simulink model "QPSK_synch_baseband"  (R2024a)
settings: Solver=VariableStepDiscrete  StartTime=0.0  StopTime=500000/fs  RelTol=1e-3  EnableMultiTasking=on
values from neighbouring files (symbols this model uses):
  fs = 50e6    (= 50000000)    [test.m]    (also in workspaceLoader.m = 75000000)
  K1 = (4*d*Bn*ts)/(Ko*Kp*(d+1/(4*d)))    (= 0.0399959725225)    [test.m]
  K2 = (4*(Bn*ts)^2)/(Ko*Kp*(d+1/4*d)^2)    (= 0.0011523480091)    [test.m]
  Ko = 1    [test.m]
undefined symbols (not defined in the file or in its folder): startfcn_constellation
libraries: dspfdesign x2, commfilt2 x2, dspsigops x2
CloseFcn:
  | closefcn_model;
Description:
  | Software, Simulation Examples and Design Exercises Licence Agreement
  | 
  | This license agreement refers to the simulation examples, design exercises and files,
  | and associated software MATLAB and Simulink resources that accompany the book:
  | 
  |      Title: Software Defined Radio using MATLAB & Simulink and the RTL-SDR
  |      Published by Strathclyde Academic Media, 2015
  |      Authored by Robert W. Stewart, Kenneth W. Barlee, Dale S.W. Atkinson,
  |      and Louise H. Crockett
  | 
  | and made available as a download from, www.desktopSDR.com or variously acquired
  | by other means such as via USB storage, cloud storage, disk or any other electronic
  | or optical or magnetic storage mechanism. These files and associated software may
  | be used subject to the terms of agreement of the conditions below:
  | 
  |     Copyright © 2015 Robert W. Stewart, Kenneth W. Barlee, Dale S.W. Atkinson,
  |     and Louise H. Crockett
  |     All rights reserved.
  | 
  | Redistribution and use in source and binary forms, with or without modification, are
  | permitted provided that the following conditions are met:
  | 
  |    1.  Redistributions of source code must retain the above copyright notice, this list of
  |         conditions and the following disclaimer.
  | 
  |    2.  Redistributions in binary form must reproduce the above copyright notice, this
  |         list of conditions and the following disclaimer in the documentation and/or other
  |         materials provided with the distribution.
  | 
  |    3.  Neither the name of the copyright holder nor the names of its contributors may
  |         be used to endorse or promote products derived from this software without
  |         specific prior written permission.
  | 
  |    4.  In all cases, the software is, and all modifications and derivatives of the
  |         software shall be, licensed to you solely for use in conjunction with The
  |         MathWorks, Inc. products and service offerings.
  | 
  | THIS SOFTWARE IS PROVIDED BY THE COPYRIGHT HOLDERS AND CONTRIBUTORS
  | "AS IS" AND ANY EXPRESS OR IMPLIED WARRANTIES, INCLUDING, BUT NOT LIMITED
  | TO, THE IMPLIED WARRANTIES OF MERCHANTABILITY AND FITNESS FOR A
  | PARTICULAR PURPOSE ARE DISCLAIMED. IN NO EVENT SHALL THE COPYRIGHT
  | HOLDER OR CONTRIBUTORS BE LIABLE FOR ANY DIRECT, INDIRECT, INCIDENTAL,
  | SPECIAL, EXEMPLARY, OR CONSEQUENTIAL DAMAGES (INCLUDING, BUT NOT
  | LIMITED TO, PROCUREMENT OF SUBSTITUTE GOODS OR SERVICES; LOSS OF USE,
  | DATA, OR PROFITS; OR BUSINESS INTERRUPTION) HOWEVER CAUSED AND ON ANY
  | THEORY OF LIABILITY, WHETHER IN CONTRACT, STRICT LIABILITY, OR TORT
  | (INCLUDING NEGLIGENCE OR OTHERWISE) ARISING IN ANY WAY OUT OF THE USE
  | OF THIS SOFTWARE, EVEN IF ADVISED OF THE POSSIBILITY OF SUCH DAMAGE.
  | 
  | 
  | Audio Tracks used in Simulations Examples and Design Exercises
  | 
  | The music and vocal files used within the Examples files and software within the book
  | were variously written, arranged, performed, recorded and produced by Garrey Rice,
  | Adam Struth, Jamie Struth, Iain Thistlethwaite and also Marshall Craigmyle who
  | collectively, and individually where appropriate, assert and retain all of their copyright,
  | performance and artistic rights. Permission to use and reproduce this music is
  | granted for all purposes associated with MATLAB and Simulink software and the
  | simulation examples and design exercises files that accompany this book. Requests to
  | use the music for any other purpose should be directed to: info@desktopSDR.com.
  | For information on music track names, full credits, and links to the musicians please
  | refer to www.desktopSDR.com/more/audio.
settings Model: Creator=desktopSDR Team  LastModifiedBy=admin
settings SolverCC: AlgebraicLoopSolver=TrustRegion
settings DataIOCC: SaveFormat=Array  SaveOutput=off  SignalLogging=off  SaveTime=off  ReturnWorkspaceOutputs=off
settings OptimizationCC: LifeSpan=inf
settings DebuggingCC: UnderspecifiedInitializationDetection=Classic  MergeDetectMultiDrivingBlocksExec=none  SolverPrmCheckMsg=warning  UnconnectedInputMsg=warning  UnconnectedOutputMsg=warning  UnconnectedLineMsg=warning  SFUnexpectedBacktrackingDiag=warning  SFNoUnconditionalDefaultTransitionDiag=warning  SFExecutionAtInitializationDiag=none  ArithmeticOperatorsInVariantConditions=warning
settings HardwareCC: ProdBitPerPointer=32  ProdBitPerSizeT=32  ProdBitPerPtrDiffT=32  ProdLargestAtomicFloat=None  ProdIntDivRoundTo=Undefined  ProdEndianess=Unspecified  ProdWordSize=32  ProdHWDeviceType=32-bit Generic
settings ModelReferenceCC: PropagateSignalLabelsOutOfModel=off
settings SFSimCC: SimUseLocalCustomCode=off  CustomCodeUndefinedFunction=UseInterfaceOnly
settings RTWCC: RTWUseLocalCustomCode=off  GPUComputeCapability=3.5
settings CodeAppCC: StateflowObjectComments=on
settings GRTTargetCC: TargetLangStandard=C89/C90 (ANSI)
settings ConfigComp: CovMetricSettings=dw  CovSaveCumulativeToWorkspaceVar=on  CovSaveSingleToWorkspaceVar=on  CovExternalEMLEnable=off  CovSFcnEnable=off

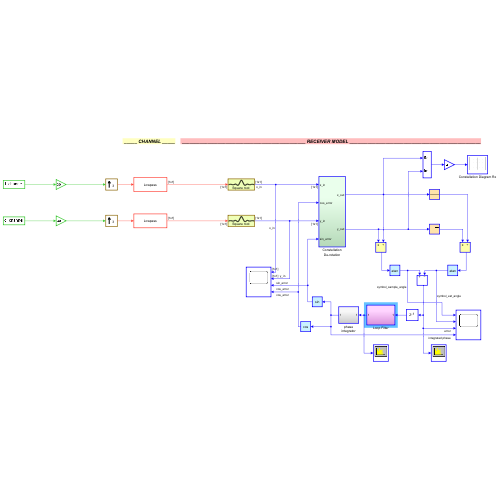
[thumbnail: Simulink's stored preview of the top-level diagram]
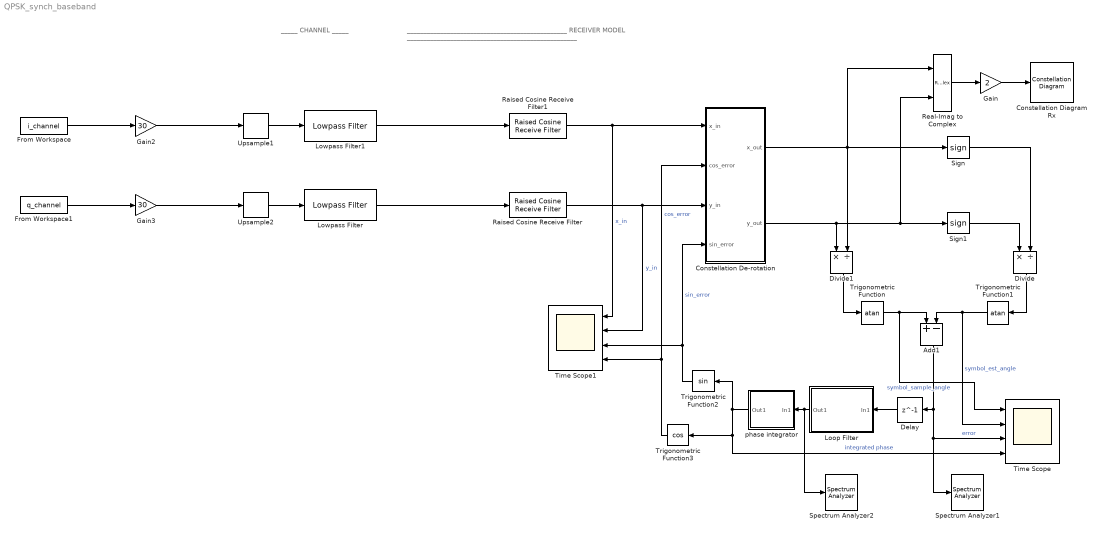
== system QPSK_synch_baseband ==
  note: _____ CHANNEL _____
  note: ________________________________________________ RECEIVER MODEL ___________________________________________________
  Add1 : Sum  Inputs=+-
  Constellation De-rotation : Subsystem
  Constellation Diagram Rx : ConstellationDiagram  StartFcn=startfcn_constellation;  WindowPosition=[141.000000,325.000000,673.000000,483.000000,]  Visible=on  ScopeFrameLocation=window  SamplesPerSymbol=2  SymbolsToDisplaySource=Property  SymbolsToDisplay=200  XLimits=[-5.052829626372052,5.889947737253722]  YLimits=[-4.966753141002106,5.071363133543149]  ColorFading=on  DefaultConfigurationName=comm.scopes.ConstellationDiagramBlockCfg
  Delay : Delay  DelayLength=1
  Divide : Product  Inputs=*/  OutMax=100000  SaturateOnIntegerOverflow=on
  Divide1 : Product  Inputs=*/  OutMax=100000  SaturateOnIntegerOverflow=on
  From Workspace : FromWorkspace  VariableName=i_channel  SampleTime=1/(fs)  Interpolate=off  OutputAfterFinalValue=Setting to zero
  From Workspace1 : FromWorkspace  VariableName=q_channel  SampleTime=1/(fs)  Interpolate=off  OutputAfterFinalValue=Setting to zero
  Gain : Gain  Gain=2
  Gain2 : Gain  Gain=30
  Gain3 : Gain  Gain=30
  Loop Filter : Subsystem
  Lowpass Filter : dspfdesign/Lowpass Filter  FilterType=FIR  DesignForMinimumOrder=off  FilterOrder=160  PassbandFrequency=23e6  StopbandFrequency=12e3  PassbandRipple=0.1  StopbandAttenuation=80  SampleRateMode=Specify on dialog  SampleRate=3*fs  SimulateUsing=Interpreted execution  roundingMode=Floor  coeffsDataTypeStr=fixdt(1,16)
  Lowpass Filter1 : dspfdesign/Lowpass Filter  FilterType=FIR  DesignForMinimumOrder=off  FilterOrder=160  PassbandFrequency=23e6  StopbandFrequency=28e6  PassbandRipple=0.1  StopbandAttenuation=80  SampleRateMode=Specify on dialog  SampleRate=fs*3  SimulateUsing=Code generation  roundingMode=Floor  coeffsDataTypeStr=fixdt(1,16)
  Raised Cosine Receive Filter : commfilt2/Raised Cosine Receive Filter  filtType=Square root  R=0.33  filtSpan=8  N=4  downFactor=4  downOffset=0  filterGain=1  RateOptions=Allow multirate processing  framing=Allow multirate processing  checkCoeff=off  variableName=rcRxFilt  currentFiltSpan=8  D=(8)/2  inputOffset=0  sampMode=Mute  saveAsFlag=0  rateMode=Downsampling  checkGain=Normalized  launchFVT=on  roundingMode=Floor  overflowMode=off  coeffDataTypeStr=Inherit: Same word length as input  coeffMin=[]  coeffMax=[]  coeffLastDataTypeStr=Inherit: Same word length as input  accumDataTypeStr=Inherit: Same as product output  accumLastDataTypeStr=Inherit: Same as product output  outputDataTypeStr=Inherit: Same as accumulator  outputMin=[]  outputMax=[]  outputLastDataTypeStr=Inherit: Same as accumulator
  Raised Cosine Receive Filter1 : commfilt2/Raised Cosine Receive Filter  filtType=Square root  R=0.33  filtSpan=8  N=4  downFactor=4  downOffset=0  filterGain=1  RateOptions=Allow multirate processing  framing=Allow multirate processing  checkCoeff=off  variableName=rcRxFilt1  currentFiltSpan=8  D=(8)/2  inputOffset=0  sampMode=Mute  saveAsFlag=0  rateMode=Downsampling  checkGain=Normalized  launchFVT=on  roundingMode=Floor  overflowMode=off  coeffDataTypeStr=Inherit: Same word length as input  coeffMin=[]  coeffMax=[]  coeffLastDataTypeStr=Inherit: Same word length as input  accumDataTypeStr=Inherit: Same as product output  accumLastDataTypeStr=Inherit: Same as product output  outputDataTypeStr=Inherit: Same as accumulator  outputMin=[]  outputMax=[]  outputLastDataTypeStr=Inherit: Same as accumulator
  Real-Imag to Complex : RealImagToComplex
  Sign : Signum
  Sign1 : Signum
  Spectrum Analyzer1 : SpectrumAnalyzer  WindowPosition=[996.000000,294.000000,800.000000,500.000000,]  Visible=on  ScopeFrameLocation=window  Span=150000000  StartFrequency=-75000000  StopFrequency=75000000  YLimits=[-11.71237975,-3.91542327]  SelectedToolstripTab=spectrumAnalyzerToolstrip.spectrumTab
  Spectrum Analyzer2 : SpectrumAnalyzer  WindowPosition=[173.000000,294.000000,800.000000,500.000000,]  Visible=on  ScopeFrameLocation=window  Span=150000000  StartFrequency=-75000000  StopFrequency=75000000  YLimits=[-44.48404203,12.65845316]  SelectedToolstripTab=spectrumAnalyzerToolstrip.spectrumTab
  Time Scope : Scope  NumInputPorts=4
      settings: StartFcn=startfcn_time_scope;
  Time Scope1 : Scope  NumInputPorts=4
      settings: StartFcn=startfcn_time_scope;
  Trigonometric Function : Trigonometry  Operator=atan  OutputSignalType=real
  Trigonometric Function1 : Trigonometry  Operator=atan  OutputSignalType=real
  Trigonometric Function2 : Trigonometry
  Trigonometric Function3 : Trigonometry  Operator=cos
  Upsample1 : dspsigops/Upsample  FactorSource=Dialog parameter  N=3  Nmax=16  phase=0  RateOptions=Allow multirate processing  ic=0  mode=Unused parameter value
  Upsample2 : dspsigops/Upsample  FactorSource=Dialog parameter  N=3  Nmax=16  phase=0  RateOptions=Allow multirate processing  ic=0  mode=Unused parameter value
  phase integrator : Subsystem
  wires:
  Real-Imag to Complex/1 -> Gain/1
  Gain/1 -> Constellation Diagram Rx/1
  Sign/1 -> Divide/2
  Sign1/1 -> Divide/1
  Trigonometric Function/1 -> Add1/1, Time Scope/1  "symbol_sample_angle"
  Trigonometric Function1/1 -> Time Scope/2, Add1/2  "symbol_est_angle"
  Loop Filter/1(Out1) -> Spectrum Analyzer2/1, phase integrator/1(In1)
  Trigonometric Function2/1 -> Time Scope1/3, Constellation De-rotation/4(sin_error)  "sin_error"
  Constellation De-rotation/2(y_out) -> Sign1/1, Real-Imag to Complex/2, Divide1/1
  Raised Cosine Receive Filter1/1 -> Time Scope1/1, Constellation De-rotation/1(x_in)  "x_in"
  Raised Cosine Receive Filter/1 -> Time Scope1/2, Constellation De-rotation/3(y_in)  "y_in"
  Trigonometric Function3/1 -> Time Scope1/4, Constellation De-rotation/2(cos_error)  "cos_error"
  Divide/1 -> Trigonometric Function1/1
  Divide1/1 -> Trigonometric Function/1
  Delay/1 -> Loop Filter/1(In1)
  Add1/1 -> Spectrum Analyzer1/1, Time Scope/3, Delay/1  "error"
  phase integrator/1(Out1) -> Trigonometric Function2/1, Time Scope/4, Trigonometric Function3/1  "integrated phase"
  Constellation De-rotation/1(x_out) -> Real-Imag to Complex/1, Sign/1, Divide1/2
  Upsample1/1 -> Lowpass Filter1/1
  Gain2/1 -> Upsample1/1
  From Workspace/1 -> Gain2/1
  From Workspace1/1 -> Gain3/1
  Gain3/1 -> Upsample2/1
  Upsample2/1 -> Lowpass Filter/1
  Lowpass Filter1/1 -> Raised Cosine Receive Filter1/1
  Lowpass Filter/1 -> Raised Cosine Receive Filter/1

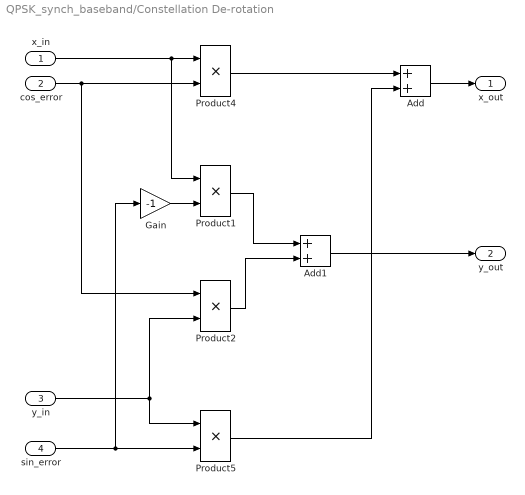
== system QPSK_synch_baseband/Constellation De-rotation ==
  x_in : Inport
  cos_error : Inport  Port=2
  y_in : Inport  Port=3
  sin_error : Inport  Port=4
  Add : Sum
  Add1 : Sum
  Gain : Gain  Gain=-1
  Product{1..2,4..5} (4 alike) : Product
  x_out : Outport
  y_out : Outport  Port=2
  wires:
  Product4/1 -> Add/1
  y_in/1 -> Product2/2, Product5/1
  sin_error/1 -> Gain/1, Product5/2
  x_in/1 -> Product1/1, Product4/1
  Product5/1 -> Add/2
  cos_error/1 -> Product2/1, Product4/2
  Add/1 -> x_out/1
  Gain/1 -> Product1/2
  Product2/1 -> Add1/2
  Product1/1 -> Add1/1
  Add1/1 -> y_out/1

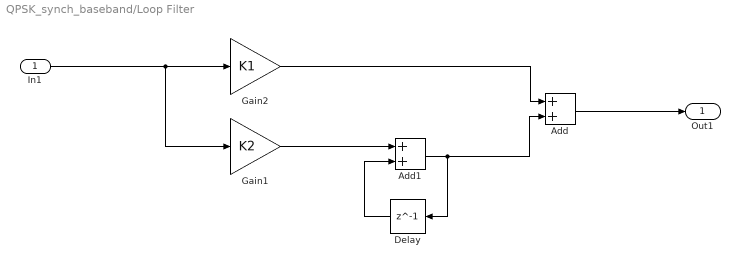
== system QPSK_synch_baseband/Loop Filter ==
  In1 : Inport
  Add : Sum
  Add1 : Sum
  Delay : Delay  DelayLength=1
  Gain1 : Gain  Gain=K2
  Gain2 : Gain  Gain=K1
  Out1 : Outport
  wires:
  Add/1 -> Out1/1
  Gain2/1 -> Add/1
  Delay/1 -> Add1/2
  Add1/1 -> Delay/1, Add/2
  Gain1/1 -> Add1/1
  In1/1 -> Gain1/1, Gain2/1

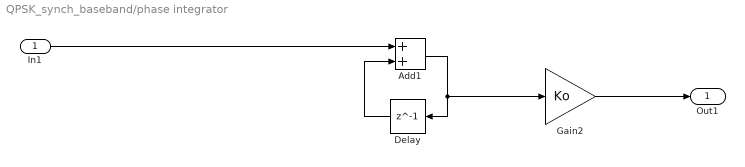
== system QPSK_synch_baseband/phase integrator ==
  In1 : Inport
  Add1 : Sum
  Delay : Delay  DelayLength=1
  Gain2 : Gain  Gain=Ko
  Out1 : Outport
  wires:
  In1/1 -> Add1/1
  Add1/1 -> Gain2/1, Delay/1
  Delay/1 -> Add1/2
  Gain2/1 -> Out1/1
